simulink model "Laborversuch_2_ab"  (R2023b)
settings: Solver=VariableStepAuto  StartTime=0.0  StopTime=30  RelTol=1e-3
values from neighbouring files (symbols this model uses):
  AB = 0.0226    [Versuch_2_parameter_c.m]
  C = 0.003    [Versuch_2_parameter_c.m]
  KR = 0.01    [Versuch_2_parameter_c.m]
settings Model: Creator=danie  LastModifiedBy=danie

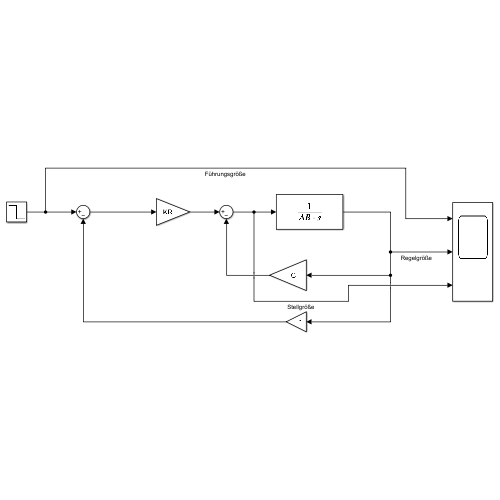
[thumbnail: Simulink's stored preview of the top-level diagram]
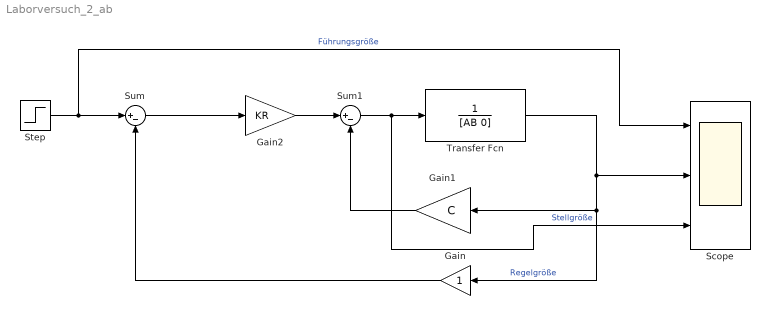
== system Laborversuch_2_ab ==
  Gain : Gain
  Gain1 : Gain  Gain=C
  Gain2 : Gain  Gain=KR
  Scope : Scope  NumInputPorts=3
  Step : Step  Time=30  Before=0.1  After=0  SampleTime=0
  Sum : Sum  Inputs=|+-
  Sum1 : Sum  Inputs=|+-
  Transfer Fcn : TransferFcn  Denominator=[AB 0]
  wires:
  Transfer Fcn/1 -> Scope/2, Gain1/1, Gain/1  "Regelgröße"
  Gain1/1 -> Sum1/2
  Gain2/1 -> Sum1/1
  Sum/1 -> Gain2/1
  Gain/1 -> Sum/2
  Step/1 -> Scope/1, Sum/1  "Führungsgröße"
  Sum1/1 -> Scope/3, Transfer Fcn/1  "Stellgröße"
